simulink model "five_tank_hybrid_system"  (R2019a)
settings: Solver=FixedStepDiscrete  StartTime=0.0  StopTime=T  FixedStep=Ts  RelTol=1e-3
InitFcn:
  | load_parameters
values from neighbouring files (symbols this model uses):
  A1u = 0.0573+0.00286    (= 0.06016)    [load_parameters.m]
  A2u = 0.0573+0.00286    (= 0.06016)    [load_parameters.m]
  A3u = 0.0346+0.0017    (= 0.0363)    [load_parameters.m]
  A4u = 0.0346+0.0017    (= 0.0363)    [load_parameters.m]
  A5u = 0.0707+0.00353    (= 0.07423)    [load_parameters.m]
  Ap1u = 3.167e-5+6.33e-6    (= 3.8e-05)    [load_parameters.m]
  Ap2u = 3.167e-5+6.33e-6    (= 3.8e-05)    [load_parameters.m]
  Ap3u = 3.167e-5+6.33e-6    (= 3.8e-05)    [load_parameters.m]
  Ap4u = 3.167e-5+6.33e-6    (= 3.8e-05)    [load_parameters.m]
  Ap5u = 3.167e-5+6.33e-6    (= 3.8e-05)    [load_parameters.m]
  Av1u = 3.167e-5+6.33e-6    (= 3.8e-05)    [load_parameters.m]
  Av2u = 3.167e-5+6.33e-6    (= 3.8e-05)    [load_parameters.m]
  Av3u = 3.167e-5+6.33e-6    (= 3.8e-05)    [load_parameters.m]
  Av4u = 3.167e-5+6.33e-6    (= 3.8e-05)    [load_parameters.m]
  cp1u = 0.68-0.0675    (= 0.6125)    [load_parameters.m]
  cp2u = 0.68-0.0675    (= 0.6125)    [load_parameters.m]
  cp3u = 0.4-0.038    (= 0.362)    [load_parameters.m]
  cp4u = 0.4-0.038    (= 0.362)    [load_parameters.m]
  cp5u = 0.7-0.068    (= 0.632)    [load_parameters.m]
  cv1u = 0.62-0.0615    (= 0.5585)    [load_parameters.m]
  cv2u = 0.62-0.0615    (= 0.5585)    [load_parameters.m]
  cv3u = 0.37-0.0365    (= 0.3335)    [load_parameters.m]
  cv4u = 0.37-0.0365    (= 0.3335)    [load_parameters.m]
  g = 9.81    [load_parameters.m]
  rho1 = 0.005    [load_parameters.m]
  rho2 = 0.005    [load_parameters.m]
  rho3 = 0.005    [load_parameters.m]
  rho4 = 0.005    [load_parameters.m]
  rho5 = 0.0063    [load_parameters.m]
  Ts = 0.01    [load_parameters.m]
  v = 0.02    [load_parameters.m]
  x1_0 = 0.3    [load_parameters.m]
  X1max = 0.4    [load_parameters.m]
  X1min = 0.1    [load_parameters.m]
  X1overflow = 0.405    [load_parameters.m]
  x2_0 = 0.12    [load_parameters.m]
  X2max = 0.4    [load_parameters.m]
  X2min = 0.1    [load_parameters.m]
  X2overflow = 0.405    [load_parameters.m]
  x3_0 = 0.15    [load_parameters.m]
  X3max = 0.35    [load_parameters.m]
  X3min = 0.1    [load_parameters.m]
  X3overflow = 0.355    [load_parameters.m]
  x4_0 = 0.3    [load_parameters.m]
  X4max = 0.35    [load_parameters.m]
  X4min = 0.1    [load_parameters.m]
  X4overflow = 0.355    [load_parameters.m]
  x5_0 = 0.09    [load_parameters.m]
  X5max = 0.2    [load_parameters.m]
  X5min = 0.05    [load_parameters.m]
  X5overflow = 0.205    [load_parameters.m]
  xi = 0.02    [load_parameters.m]
undefined symbols (not defined in the file or in its folder): dfilt, DiscIntNeverNeededParam
libraries: dsparch4 x5
(part 1 of 2)
settings Model: Creator=Constantinos  LastModifiedBy=Constantinos
settings DataIOCC: ReturnWorkspaceOutputs=off
settings DebuggingCC: PregeneratedLibrarySubsystemCodeDiagnostic=none  ArithmeticOperatorsInVariantConditions=warning
settings SFSimCC: SimUseLocalCustomCode=off
settings RTWCC: RTWUseLocalCustomCode=off

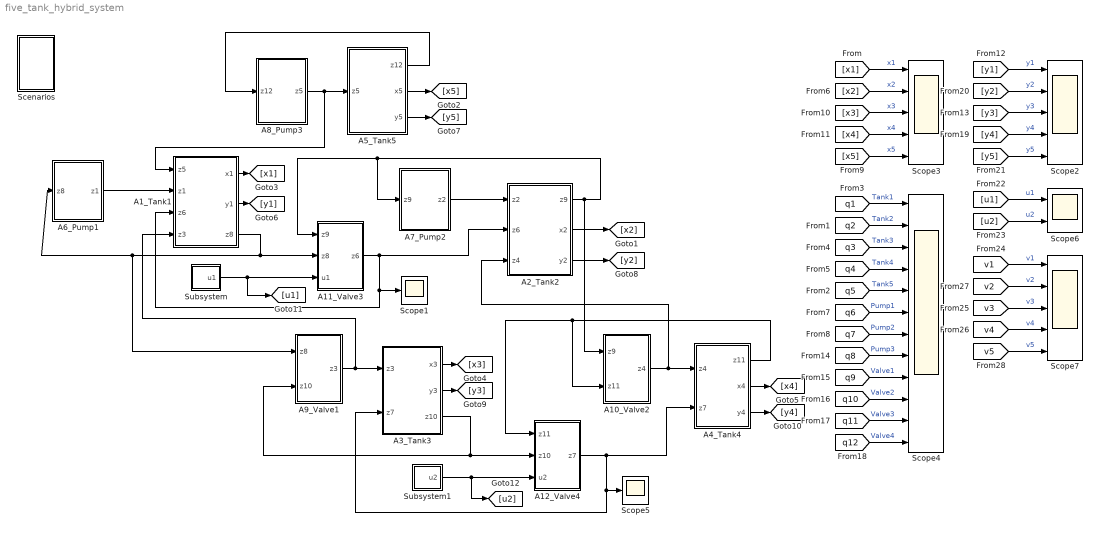
== system five_tank_hybrid_system ==
  A10_Valve2 : Subsystem
  A11_Valve3 : Subsystem
  A12_Valve4 : Subsystem
  A1_Tank1 : Subsystem
  A2_Tank2 : Subsystem
  A3_Tank3 : Subsystem
  A4_Tank4 : Subsystem
  A5_Tank5 : Subsystem
  A6_Pump1 : Subsystem
  A7_Pump2 : Subsystem
  A8_Pump3 : Subsystem
  A9_Valve1 : Subsystem
  Scenarios : Subsystem
  Scope1 : Scope
  Scope2 : Scope  NumInputPorts=5
  Scope3 : Scope  NumInputPorts=5
  Scope4 : Scope  NumInputPorts=12
  Scope5 : Scope
  Scope6 : Scope  NumInputPorts=2
  Scope7 : Scope  NumInputPorts=5
  Subsystem : Subsystem
  Subsystem1 : Subsystem
  wires:
  A6_Pump1/1(z1) -> A1_Tank1/2(z1)
  A7_Pump2/1(z2) -> A2_Tank2/1(z2)
  A8_Pump3/1(z5) -> A1_Tank1/1(z5), A5_Tank5/1(z5)
  A5_Tank5/1(z12) -> A8_Pump3/1(z12)
  A1_Tank1/3(z8) -> A6_Pump1/1(z8), A9_Valve1/1(z8), A11_Valve3/2(z8)
  A11_Valve3/1(z6) -> A2_Tank2/2(z6), Scope1/1, A1_Tank1/3(z6)
  A2_Tank2/1(z9) -> A7_Pump2/1(z9), A11_Valve3/1(z9), A10_Valve2/1(z9)
  A3_Tank3/3(z10) -> A12_Valve4/2(z10), A9_Valve1/2(z10)
  A12_Valve4/1(z7) -> Scope5/1, A3_Tank3/2(z7), A4_Tank4/2(z7)
  A4_Tank4/1(z11) -> A12_Valve4/1(z11), A10_Valve2/2(z11)
  A9_Valve1/1(z3) -> A1_Tank1/4(z3), A3_Tank3/1(z3)
  A10_Valve2/1(z4) -> A2_Tank2/3(z4), A4_Tank4/1(z4)
  A5_Tank5/2(x5) -> [x5]
  [q1] -> Scope4/1  "Tank1"
  [x4] -> Scope3/4  "x4"
  [q6] -> Scope4/6  "Pump1"
  [q4] -> Scope4/4  "Tank4"
  [x2] -> Scope3/2  "x2"
  [q5] -> Scope4/5  "Tank5"
  [q2] -> Scope4/2  "Tank2"
  [q9] -> Scope4/9  "Valve1"
  [q12] -> Scope4/12  "Valve4"
  [q3] -> Scope4/3  "Tank3"
  [x3] -> Scope3/3  "x3"
  [x1] -> Scope3/1  "x1"
  [q10] -> Scope4/10  "Valve2"
  [q8] -> Scope4/8  "Pump3"
  [q11] -> Scope4/11  "Valve3"
  [q7] -> Scope4/7  "Pump2"
  A2_Tank2/2(x2) -> [x2]
  A1_Tank1/1(x1) -> [x1]
  A3_Tank3/1(x3) -> [x3]
  A4_Tank4/2(x4) -> [x4]
  A1_Tank1/2(y1) -> [y1]
  [y1] -> Scope2/1  "y1"
  [y5] -> Scope2/5  "y5"
  [y3] -> Scope2/3  "y3"
  [y2] -> Scope2/2  "y2"
  [y4] -> Scope2/4  "y4"
  A5_Tank5/3(y5) -> [y5]
  A2_Tank2/3(y2) -> [y2]
  A3_Tank3/2(y3) -> [y3]
  A4_Tank4/3(y4) -> [y4]
  [x5] -> Scope3/5  "x5"
  [u1] -> Scope6/1  "u1"
  [u2] -> Scope6/2  "u2"
  [v4] -> Scope7/4  "v4"
  [v2] -> Scope7/2  "v2"
  [v3] -> Scope7/3  "v3"
  [v5] -> Scope7/5  "v5"
  [v1] -> Scope7/1  "v1"
  Subsystem1/1(u2) -> [u2], A12_Valve4/3(u2)
  Subsystem/1(u1) -> [u1], A11_Valve3/3(u1)

== system five_tank_hybrid_system/A10_Valve2 ==
  z9 : Inport
  z11 : Inport  Port=2
  Chart : Stateflow chart  TreatAsAtomicUnit=on
  Constant1 : Constant  Value=0
  Constant3 : Constant  Value=cv2u
  Constant4 : Constant  Value=Av2u
  Constant5 : Constant  Value=g
  Index Vector : MultiPortSwitch  DataPortOrder=Specify indices  Inputs=1  DataPortIndices={1,2,3,4}
  MATLAB Function : MATLAB Function  TreatAsAtomicUnit=on
  z4 : Outport
  tag scope: q10=global
  wires:
  Index Vector/1 -> z4/1
  [phi12] -> Chart/3(phi12)
  [phi11] -> Chart/2(phi11)
  MATLAB Function/1(z) -> Index Vector/3, Index Vector/5
  Constant4/1 -> MATLAB Function/2(Av)
  Constant5/1 -> MATLAB Function/4(g)
  z11/1 -> Chart/1(x4)
  Constant3/1 -> MATLAB Function/1(cv)
  Chart/1(q) -> [q10], Index Vector/1
  Constant1/1 -> Index Vector/4, Index Vector/2
  z9/1 -> MATLAB Function/3(in1)

== system five_tank_hybrid_system/A11_Valve3 ==
  z9 : Inport
  z8 : Inport  Port=2
  u1 : Inport  Port=3
  Chart : Stateflow chart  TreatAsAtomicUnit=on
  Constant1 : Constant  Value=0
  Constant3 : Constant  Value=cv3u
  Constant4 : Constant  Value=Av3u
  Constant5 : Constant  Value=g
  Index Vector : MultiPortSwitch  DataPortOrder=Specify indices  Inputs=1  DataPortIndices={1,2,3,4}
  MATLAB Function : MATLAB Function  TreatAsAtomicUnit=on
  z6 : Outport
  tag scope: q11=global
  wires:
  z9/1 -> MATLAB Function/4(in2)
  Constant3/1 -> MATLAB Function/1(cv)
  z8/1 -> MATLAB Function/3(in1)
  Constant5/1 -> MATLAB Function/5(g)
  Constant4/1 -> MATLAB Function/2(Av)
  MATLAB Function/1(z) -> Index Vector/3, Index Vector/5
  Chart/1(q) -> [q11], Index Vector/1
  [phi13] -> Chart/2(phi13)
  [phi14] -> Chart/3(phi14)
  Index Vector/1 -> z6/1
  u1/1 -> Chart/1(u1)
  Constant1/1 -> Index Vector/4, Index Vector/2

== system five_tank_hybrid_system/A12_Valve4 ==
  z11 : Inport
  z10 : Inport  Port=2
  u2 : Inport  Port=3
  Chart : Stateflow chart  TreatAsAtomicUnit=on
  Constant2 : Constant  Value=0
  Constant3 : Constant  Value=cv4u
  Constant4 : Constant  Value=Av4u
  Constant5 : Constant  Value=g
  Index Vector : MultiPortSwitch  DataPortOrder=Specify indices  Inputs=1  DataPortIndices={1,2,3,4}
  MATLAB Function : MATLAB Function  TreatAsAtomicUnit=on
  z7 : Outport
  tag scope: q12=global
  wires:
  u2/1 -> Chart/1(u2)
  Index Vector/1 -> z7/1
  [phi16] -> Chart/3(phi16)
  [phi15] -> Chart/2(phi15)
  Chart/1(q) -> [q12], Index Vector/1
  MATLAB Function/1(z) -> Index Vector/3, Index Vector/5
  Constant4/1 -> MATLAB Function/2(Av)
  Constant5/1 -> MATLAB Function/5(g)
  Constant2/1 -> Index Vector/2, Index Vector/4
  z10/1 -> MATLAB Function/3(in1)
  Constant3/1 -> MATLAB Function/1(cv)
  z11/1 -> MATLAB Function/4(in2)

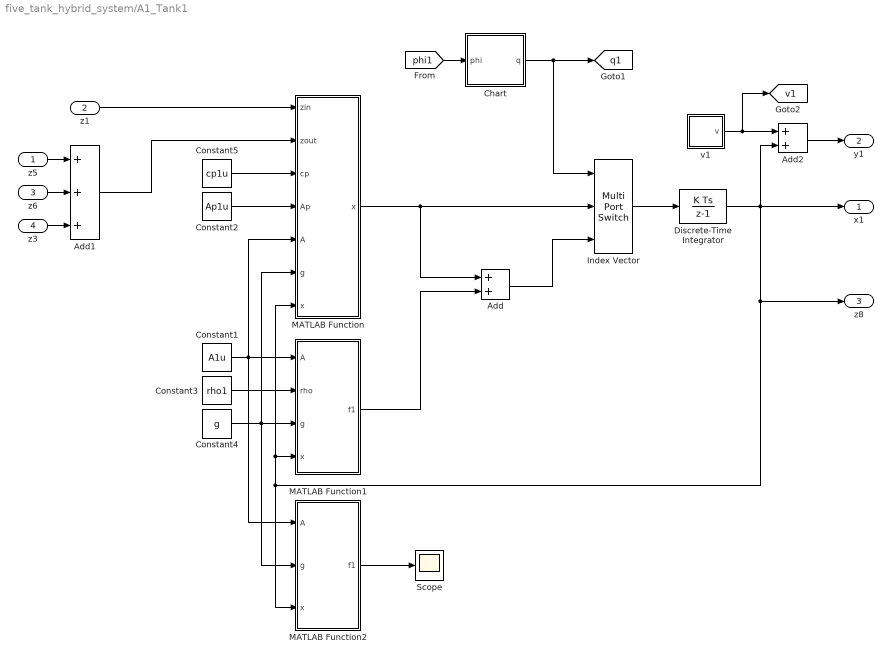
== system five_tank_hybrid_system/A1_Tank1 ==
  z5 : Inport
  z1 : Inport  Port=2
  z6 : Inport  Port=3
  z3 : Inport  Port=4
  Add : Sum
  Add1 : Sum  Inputs=+++
  Add2 : Sum
  Chart : Stateflow chart  TreatAsAtomicUnit=on
  Constant1 : Constant  Value=A1u
  Constant2 : Constant  Value=Ap1u
  Constant3 : Constant  Value=rho1
  Constant4 : Constant  Value=g
  Constant5 : Constant  Value=cp1u
  Discrete-Time Integrator : DiscreteIntegrator  InitialCondition=x1_0  SampleTime=-1  LimitOutput=on  UpperSaturationLimit=X1overflow  LowerSaturationLimit=0  ICPrevOutput=DiscIntNeverNeededParam  ICPrevScaledInput=DiscIntNeverNeededParam
  Index Vector : MultiPortSwitch  DataPortOrder=Specify indices  Inputs=1  DataPortIndices={1,2}
  MATLAB Function : MATLAB Function  TreatAsAtomicUnit=on
  MATLAB Function1 : MATLAB Function  TreatAsAtomicUnit=on
  MATLAB Function2 : MATLAB Function  TreatAsAtomicUnit=on
  Scope : Scope
  v1 : Subsystem
  x1 : Outport
  y1 : Outport  Port=2
  z8 : Outport  Port=3
  tag scope: q1=global, v1=global
  wires:
  Index Vector/1 -> Discrete-Time Integrator/1
  Add/1 -> Index Vector/3
  MATLAB Function/1(x) -> Add/1, Index Vector/2
  MATLAB Function1/1(f1) -> Add/2
  Discrete-Time Integrator/1 -> Add2/2, x1/1, MATLAB Function2/3(x), MATLAB Function/7("x "), MATLAB Function1/4(x), z8/1
  Constant5/1 -> MATLAB Function/3(cp)
  Constant2/1 -> MATLAB Function/4(Ap)
  Constant1/1 -> MATLAB Function2/1(A), MATLAB Function/5(A), MATLAB Function1/1(A)
  Constant3/1 -> MATLAB Function1/2(rho)
  Constant4/1 -> MATLAB Function2/2(g), MATLAB Function/6(g), MATLAB Function1/3(g)
  z1/1 -> MATLAB Function/1(zin)
  z3/1 -> Add1/3
  z6/1 -> Add1/2
  z5/1 -> Add1/1
  Add1/1 -> MATLAB Function/2(zout)
  Chart/1(q) -> [q1], Index Vector/1
  [phi1] -> Chart/1(phi)
  v1/1(v) -> [v1], Add2/1
  Add2/1 -> y1/1
  MATLAB Function2/1(f1) -> Scope/1

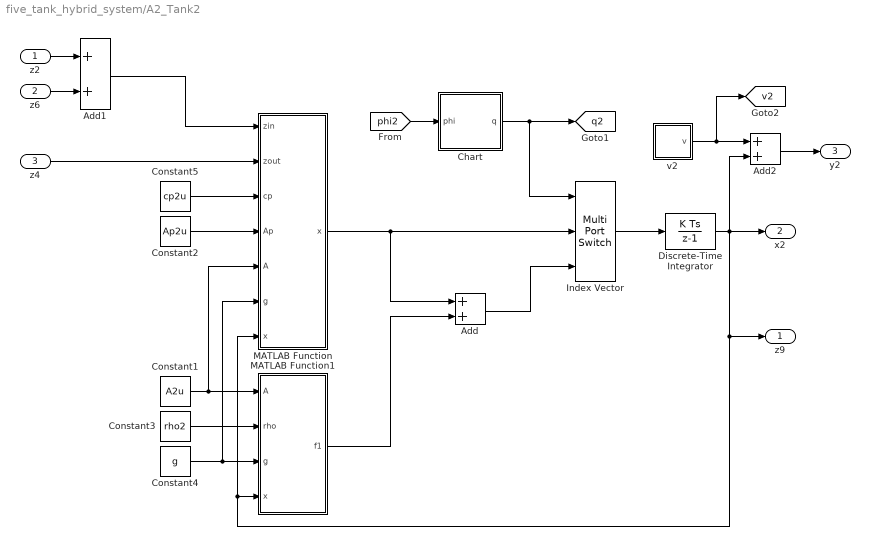
== system five_tank_hybrid_system/A2_Tank2 ==
  z2 : Inport
  z6 : Inport  Port=2
  z4 : Inport  Port=3
  Add : Sum
  Add1 : Sum
  Add2 : Sum
  Chart : Stateflow chart  TreatAsAtomicUnit=on
  Constant1 : Constant  Value=A2u
  Constant2 : Constant  Value=Ap2u
  Constant3 : Constant  Value=rho2
  Constant4 : Constant  Value=g
  Constant5 : Constant  Value=cp2u
  Discrete-Time Integrator : DiscreteIntegrator  InitialCondition=x2_0  SampleTime=-1  LimitOutput=on  UpperSaturationLimit=X2overflow  LowerSaturationLimit=0  ICPrevOutput=DiscIntNeverNeededParam  ICPrevScaledInput=DiscIntNeverNeededParam
  Index Vector : MultiPortSwitch  DataPortOrder=Specify indices  Inputs=1  DataPortIndices={1,2}
  MATLAB Function : MATLAB Function  TreatAsAtomicUnit=on
  MATLAB Function1 : MATLAB Function  TreatAsAtomicUnit=on
  v2 : Subsystem
  z9 : Outport
  x2 : Outport  Port=2
  y2 : Outport  Port=3
  tag scope: q2=global, v2=global
  wires:
  Constant4/1 -> MATLAB Function/6(g), MATLAB Function1/3(g)
  Constant3/1 -> MATLAB Function1/2(rho)
  Constant1/1 -> MATLAB Function1/1(A), MATLAB Function/5(A)
  Constant2/1 -> MATLAB Function/4(Ap)
  Constant5/1 -> MATLAB Function/3(cp)
  MATLAB Function1/1(f1) -> Add/2
  MATLAB Function/1(x) -> Index Vector/2, Add/1
  Add/1 -> Index Vector/3
  Index Vector/1 -> Discrete-Time Integrator/1
  [phi2] -> Chart/1(phi)
  Chart/1(q) -> [q2], Index Vector/1
  Discrete-Time Integrator/1 -> Add2/2, x2/1, z9/1, MATLAB Function/7("x "), MATLAB Function1/4(x)
  Add2/1 -> y2/1
  v2/1(v) -> [v2], Add2/1
  Add1/1 -> MATLAB Function/1(zin)
  z2/1 -> Add1/1
  z6/1 -> Add1/2
  z4/1 -> MATLAB Function/2(zout)

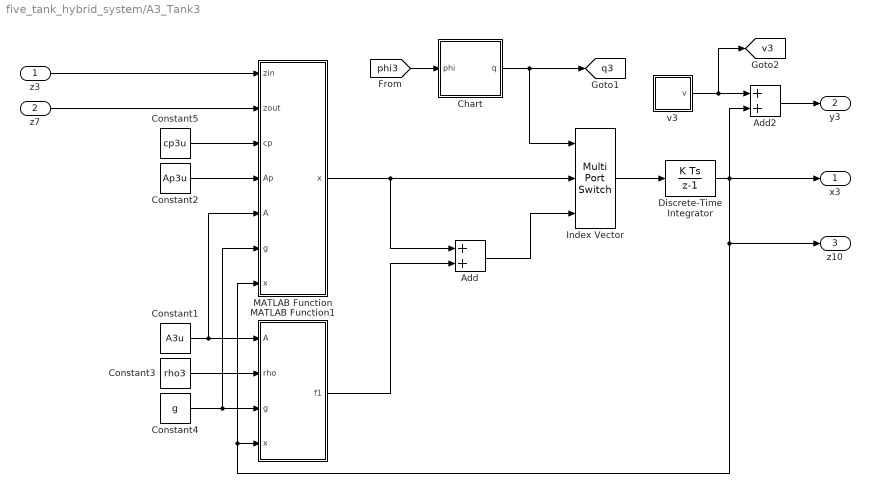
== system five_tank_hybrid_system/A3_Tank3 ==
  z3 : Inport
  z7 : Inport  Port=2
  Add : Sum
  Add2 : Sum
  Chart : Stateflow chart  TreatAsAtomicUnit=on
  Constant1 : Constant  Value=A3u
  Constant2 : Constant  Value=Ap3u
  Constant3 : Constant  Value=rho3
  Constant4 : Constant  Value=g
  Constant5 : Constant  Value=cp3u
  Discrete-Time Integrator : DiscreteIntegrator  InitialCondition=x3_0  SampleTime=-1  LimitOutput=on  UpperSaturationLimit=X3overflow  LowerSaturationLimit=0  ICPrevOutput=DiscIntNeverNeededParam  ICPrevScaledInput=DiscIntNeverNeededParam
  Index Vector : MultiPortSwitch  DataPortOrder=Specify indices  Inputs=1  DataPortIndices={1,2}
  MATLAB Function : MATLAB Function  TreatAsAtomicUnit=on
  MATLAB Function1 : MATLAB Function  TreatAsAtomicUnit=on
  v3 : Subsystem
  x3 : Outport
  y3 : Outport  Port=2
  z10 : Outport  Port=3
  tag scope: q3=global, v3=global
  wires:
  Chart/1(q) -> [q3], Index Vector/1
  [phi3] -> Chart/1(phi)
  Index Vector/1 -> Discrete-Time Integrator/1
  Add/1 -> Index Vector/3
  MATLAB Function/1(x) -> Add/1, Index Vector/2
  MATLAB Function1/1(f1) -> Add/2
  Constant5/1 -> MATLAB Function/3(cp)
  Constant2/1 -> MATLAB Function/4(Ap)
  Constant1/1 -> MATLAB Function/5(A), MATLAB Function1/1(A)
  Constant3/1 -> MATLAB Function1/2(rho)
  Constant4/1 -> MATLAB Function1/3(g), MATLAB Function/6(g)
  z3/1 -> MATLAB Function/1(zin)
  z7/1 -> MATLAB Function/2(zout)
  v3/1(v) -> [v3], Add2/1
  Discrete-Time Integrator/1 -> Add2/2, x3/1, MATLAB Function1/4(x), MATLAB Function/7("x "), z10/1
  Add2/1 -> y3/1

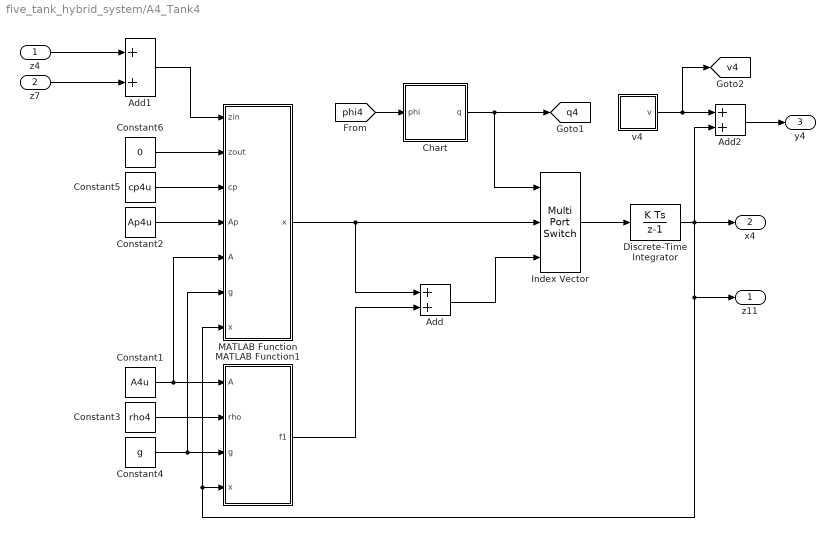
== system five_tank_hybrid_system/A4_Tank4 ==
  z4 : Inport
  z7 : Inport  Port=2
  Add : Sum
  Add1 : Sum
  Add2 : Sum
  Chart : Stateflow chart  TreatAsAtomicUnit=on
  Constant1 : Constant  Value=A4u
  Constant2 : Constant  Value=Ap4u
  Constant3 : Constant  Value=rho4
  Constant4 : Constant  Value=g
  Constant5 : Constant  Value=cp4u
  Constant6 : Constant  Value=0
  Discrete-Time Integrator : DiscreteIntegrator  InitialCondition=x4_0  SampleTime=-1  LimitOutput=on  UpperSaturationLimit=X4overflow  LowerSaturationLimit=0  ICPrevOutput=DiscIntNeverNeededParam  ICPrevScaledInput=DiscIntNeverNeededParam
  Index Vector : MultiPortSwitch  DataPortOrder=Specify indices  Inputs=1  DataPortIndices={1,2}
  MATLAB Function : MATLAB Function  TreatAsAtomicUnit=on
  MATLAB Function1 : MATLAB Function  TreatAsAtomicUnit=on
  v4 : Subsystem
  z11 : Outport
  x4 : Outport  Port=2
  y4 : Outport  Port=3
  tag scope: q4=global, v4=global
  wires:
  z4/1 -> Add1/1
  Constant4/1 -> MATLAB Function/6(g), MATLAB Function1/3(g)
  Constant3/1 -> MATLAB Function1/2(rho)
  Constant1/1 -> MATLAB Function1/1(A), MATLAB Function/5(A)
  Constant2/1 -> MATLAB Function/4(Ap)
  Constant5/1 -> MATLAB Function/3(cp)
  MATLAB Function1/1(f1) -> Add/2
  MATLAB Function/1(x) -> Index Vector/2, Add/1
  Add/1 -> Index Vector/3
  Index Vector/1 -> Discrete-Time Integrator/1
  [phi4] -> Chart/1(phi)
  Chart/1(q) -> [q4], Index Vector/1
  v4/1(v) -> [v4], Add2/1
  Discrete-Time Integrator/1 -> Add2/2, x4/1, MATLAB Function/7("x "), MATLAB Function1/4(x), z11/1
  Add2/1 -> y4/1
  Add1/1 -> MATLAB Function/1(zin)
  z7/1 -> Add1/2
  Constant6/1 -> MATLAB Function/2(zout)

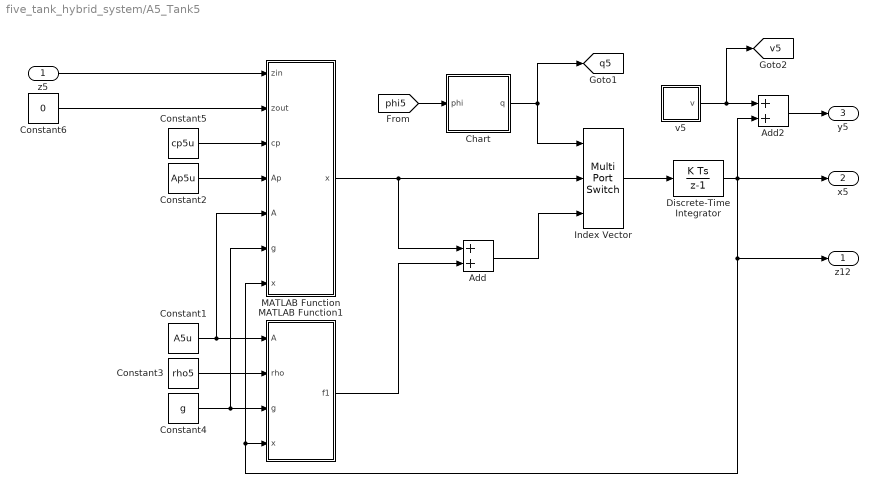
== system five_tank_hybrid_system/A5_Tank5 ==
  z5 : Inport
  Add : Sum
  Add2 : Sum
  Chart : Stateflow chart  TreatAsAtomicUnit=on
  Constant1 : Constant  Value=A5u
  Constant2 : Constant  Value=Ap5u
  Constant3 : Constant  Value=rho5
  Constant4 : Constant  Value=g
  Constant5 : Constant  Value=cp5u
  Constant6 : Constant  Value=0
  Discrete-Time Integrator : DiscreteIntegrator  InitialCondition=x5_0  SampleTime=-1  LimitOutput=on  UpperSaturationLimit=X5overflow  LowerSaturationLimit=0  ICPrevOutput=DiscIntNeverNeededParam  ICPrevScaledInput=DiscIntNeverNeededParam
  Index Vector : MultiPortSwitch  DataPortOrder=Specify indices  Inputs=1  DataPortIndices={1,2}
  MATLAB Function : MATLAB Function  TreatAsAtomicUnit=on
  MATLAB Function1 : MATLAB Function  TreatAsAtomicUnit=on
  v5 : Subsystem
  z12 : Outport
  x5 : Outport  Port=2
  y5 : Outport  Port=3
  tag scope: q5=global, v5=global
  wires:
  Chart/1(q) -> [q5], Index Vector/1
  [phi5] -> Chart/1(phi)
  Index Vector/1 -> Discrete-Time Integrator/1
  Add/1 -> Index Vector/3
  MATLAB Function/1(x) -> Add/1, Index Vector/2
  MATLAB Function1/1(f1) -> Add/2
  Constant5/1 -> MATLAB Function/3(cp)
  Constant2/1 -> MATLAB Function/4(Ap)
  Constant1/1 -> MATLAB Function/5(A), MATLAB Function1/1(A)
  Constant3/1 -> MATLAB Function1/2(rho)
  Constant4/1 -> MATLAB Function1/3(g), MATLAB Function/6(g)
  z5/1 -> MATLAB Function/1(zin)
  Constant6/1 -> MATLAB Function/2(zout)
  Discrete-Time Integrator/1 -> Add2/2, x5/1, z12/1, MATLAB Function1/4(x), MATLAB Function/7("x ")
  Add2/1 -> y5/1
  v5/1(v) -> [v5], Add2/1

== system five_tank_hybrid_system/A6_Pump1 ==
  z8 : Inport
  Chart : Stateflow chart  TreatAsAtomicUnit=on
  Clock : Clock
  Constant : Constant  Value=0
  Fcn : Fcn  Expr=0.5e-5*sin(0.1*u)+1.8e-4
  Index Vector : MultiPortSwitch  DataPortOrder=Specify indices  Inputs=1
  z1 : Outport
  tag scope: q6=global
  wires:
  [phi6] -> Chart/2(phi6)
  Clock/1 -> Fcn/1
  z8/1 -> Chart/1(x1)
  Fcn/1 -> Index Vector/3
  Constant/1 -> Index Vector/4, Index Vector/2
  Chart/1(q) -> [q6], Index Vector/1
  Index Vector/1 -> z1/1

== system five_tank_hybrid_system/A7_Pump2 ==
  z9 : Inport
  Chart1 : Stateflow chart  TreatAsAtomicUnit=on
  Clock1 : Clock
  Constant1 : Constant  Value=0
  Fcn1 : Fcn  Expr=0.5e-5*sin(0.1*u)+1.8e-4
  Index Vector1 : MultiPortSwitch  DataPortOrder=Specify indices  Inputs=1
  z2 : Outport
  tag scope: q7=global
  wires:
  Clock1/1 -> Fcn1/1
  [phi7] -> Chart1/2(phi7)
  z9/1 -> Chart1/1(x2)
  Constant1/1 -> Index Vector1/4, Index Vector1/2
  Fcn1/1 -> Index Vector1/3
  Index Vector1/1 -> z2/1
  Chart1/1(q) -> [q7], Index Vector1/1

== system five_tank_hybrid_system/A8_Pump3 ==
  z12 : Inport
  Chart2 : Stateflow chart  TreatAsAtomicUnit=on
  Clock1 : Clock
  Constant1 : Constant  Value=0
  Fcn1 : Fcn  Expr=0.5e-5*sin(0.1*u)+0.85e-4
  Index Vector1 : MultiPortSwitch  DataPortOrder=Specify indices  Inputs=1
  z5 : Outport
  tag scope: q8=global
  wires:
  Index Vector1/1 -> z5/1
  [phi8] -> Chart2/2(phi8)
  Chart2/1(q) -> [q8], Index Vector1/1
  z12/1 -> Chart2/1(x5)
  Constant1/1 -> Index Vector1/4, Index Vector1/2
  Fcn1/1 -> Index Vector1/3
  Clock1/1 -> Fcn1/1

== system five_tank_hybrid_system/A9_Valve1 ==
  z8 : Inport
  z10 : Inport  Port=2
  Chart : Stateflow chart  TreatAsAtomicUnit=on
  Constant1 : Constant  Value=0
  Constant3 : Constant  Value=cv1u
  Constant4 : Constant  Value=Av1u
  Constant5 : Constant  Value=g
  Index Vector : MultiPortSwitch  DataPortOrder=Specify indices  Inputs=1  DataPortIndices={1,2,3,4}
  MATLAB Function : MATLAB Function  TreatAsAtomicUnit=on
  z3 : Outport
  tag scope: q9=global
  wires:
  Constant3/1 -> MATLAB Function/1(cv)
  z10/1 -> Chart/1(x3)
  Constant5/1 -> MATLAB Function/4(g)
  Constant4/1 -> MATLAB Function/2(Av)
  MATLAB Function/1(z) -> Index Vector/3, Index Vector/5
  Chart/1(q) -> [q9], Index Vector/1
  [phi9] -> Chart/2(phi9)
  [phi10] -> Chart/3(phi10)
  Index Vector/1 -> z3/1
  Constant1/1 -> Index Vector/4, Index Vector/2
  z8/1 -> MATLAB Function/3(in1)

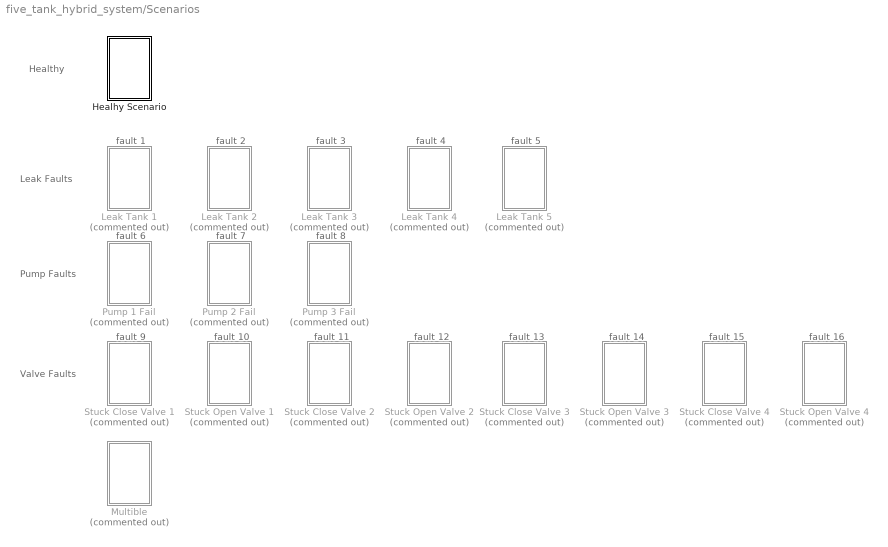
== system five_tank_hybrid_system/Scenarios ==
  note: fault 1
  note: Healthy
  note: Leak Faults
  note: Pump Faults
  note: Valve Faults
  note: fault 2
  note: fault 3
  note: fault 4
  note: fault 5
  note: fault 6
  note: fault 7
  note: fault 8
  note: fault 9
  note: fault 13
  note: fault 10
  note: fault 14
  note: fault 11
  note: fault 15
  note: fault 12
  note: fault 16
  Healhy Scenario : Subsystem
  Leak Tank 1 : Subsystem  Commented=on
  Leak Tank 2 : Subsystem  Commented=on
  Leak Tank 3 : Subsystem  Commented=on
  Leak Tank 4 : Subsystem  Commented=on
  Leak Tank 5 : Subsystem  Commented=on
  Multible : Subsystem  Commented=on
  Pump 1 Fail : Subsystem  Commented=on
  Pump 2 Fail : Subsystem  Commented=on
  Pump 3 Fail : Subsystem  Commented=on
  Stuck Close Valve 1 : Subsystem  Commented=on
  Stuck Close Valve 2 : Subsystem  Commented=on
  Stuck Close Valve 3 : Subsystem  Commented=on
  Stuck Close Valve 4 : Subsystem  Commented=on
  Stuck Open Valve 1 : Subsystem  Commented=on
  Stuck Open Valve 2 : Subsystem  Commented=on
  Stuck Open Valve 3 : Subsystem  Commented=on
  Stuck Open Valve 4 : Subsystem  Commented=on

== system five_tank_hybrid_system/Subsystem ==
  Chart : Stateflow chart  TreatAsAtomicUnit=on
  u1 : Outport
  wires:
  Chart/1(u1) -> u1/1

== system five_tank_hybrid_system/Subsystem1 ==
  Chart : Stateflow chart  TreatAsAtomicUnit=on
  u2 : Outport
  wires:
  Chart/1(u2) -> u2/1

== system five_tank_hybrid_system/A1_Tank1/v1 ==
  Highpass085 : dsparch4/Biquad Filter  Tag=BlockMethodSubSystem  FilterSource=Dialog parameters  CoeffSource=Specify via dialog  FilterObject=dfilt.df2tsos([1 0.3 0.4],[1 0.1 0.2])  IIRFiltStruct=Direct form II  BiQuadCoeffs=[1 -2 1 1 1.6638470300298394 0.8673791772124948;1 -2 1 1 1.4774912143044396 0.65822715568812495;1 -2 1 1 1.3489677452527944 0.51398189421967577;1 -2 1 1 1.2687805392030125 0.42398568894741273;1 -2 1 1 1.2303311697764827 0.38083295281952212]  ScaleValues=[0.050883036795663916;0.045183985345921322;0.041253537241720324;0.038801287436100056;0.037625445760759803;1]  IC=0  ICnum=0  ICden=0  a0Flag=Warning  optimizeScaleValues=on  ScaleValueMode=Specify via input port (g)  InputProcessing=Columns as channels (frame based)  roundingMode=Floor  overflowMode=off  scaleValueFracLength=14  denProdOutputFracLength=30  denAccumFracLength=30  secondMemoryFracLength=15
      settings: SourceProductName=DSP System Toolbox
  Saturation : Saturate  UpperLimit=xi  LowerLimit=-xi
  Scope1 : Scope
  Scope2 : Scope
  noise : UniformRandomNumber  Minimum=-v  Maximum=v  Seed=15  SampleTime=Ts
  v : Outport
  wires:
  noise/1 -> Scope1/1, Highpass085/1
  Highpass085/1 -> Scope2/1, Saturation/1
  Saturation/1 -> v/1

== system five_tank_hybrid_system/A2_Tank2/v2 ==
  Highpass085 : dsparch4/Biquad Filter  Tag=BlockMethodSubSystem  FilterSource=Dialog parameters  CoeffSource=Specify via dialog  FilterObject=dfilt.df2tsos([1 0.3 0.4],[1 0.1 0.2])  IIRFiltStruct=Direct form II  BiQuadCoeffs=[1 -2 1 1 1.6638470300298394 0.8673791772124948;1 -2 1 1 1.4774912143044396 0.65822715568812495;1 -2 1 1 1.3489677452527944 0.51398189421967577;1 -2 1 1 1.2687805392030125 0.42398568894741273;1 -2 1 1 1.2303311697764827 0.38083295281952212]  ScaleValues=[0.050883036795663916;0.045183985345921322;0.041253537241720324;0.038801287436100056;0.037625445760759803;1]  IC=0  ICnum=0  ICden=0  a0Flag=Warning  optimizeScaleValues=on  ScaleValueMode=Specify via input port (g)  InputProcessing=Columns as channels (frame based)  roundingMode=Floor  overflowMode=off  scaleValueFracLength=14  denProdOutputFracLength=30  denAccumFracLength=30  secondMemoryFracLength=15
      settings: SourceProductName=DSP System Toolbox
  Saturation : Saturate  UpperLimit=xi  LowerLimit=-xi
  Scope1 : Scope
  Scope2 : Scope
  noise : UniformRandomNumber  Minimum=-v  Maximum=v  Seed=11  SampleTime=Ts
  v : Outport
  wires:
  noise/1 -> Scope1/1, Highpass085/1
  Highpass085/1 -> Scope2/1, Saturation/1
  Saturation/1 -> v/1

== system five_tank_hybrid_system/A3_Tank3/v3 ==
  Highpass085 : dsparch4/Biquad Filter  Tag=BlockMethodSubSystem  FilterSource=Dialog parameters  CoeffSource=Specify via dialog  FilterObject=dfilt.df2tsos([1 0.3 0.4],[1 0.1 0.2])  IIRFiltStruct=Direct form II  BiQuadCoeffs=[1 -2 1 1 1.6638470300298394 0.8673791772124948;1 -2 1 1 1.4774912143044396 0.65822715568812495;1 -2 1 1 1.3489677452527944 0.51398189421967577;1 -2 1 1 1.2687805392030125 0.42398568894741273;1 -2 1 1 1.2303311697764827 0.38083295281952212]  ScaleValues=[0.050883036795663916;0.045183985345921322;0.041253537241720324;0.038801287436100056;0.037625445760759803;1]  IC=0  ICnum=0  ICden=0  a0Flag=Warning  optimizeScaleValues=on  ScaleValueMode=Specify via input port (g)  InputProcessing=Columns as channels (frame based)  roundingMode=Floor  overflowMode=off  scaleValueFracLength=14  denProdOutputFracLength=30  denAccumFracLength=30  secondMemoryFracLength=15
      settings: SourceProductName=DSP System Toolbox
  Saturation : Saturate  UpperLimit=xi  LowerLimit=-xi
  Scope1 : Scope
  Scope2 : Scope
  noise : UniformRandomNumber  Minimum=-v  Maximum=v  Seed=7  SampleTime=Ts
  v : Outport
  wires:
  noise/1 -> Scope1/1, Highpass085/1
  Highpass085/1 -> Scope2/1, Saturation/1
  Saturation/1 -> v/1

== system five_tank_hybrid_system/A4_Tank4/v4 ==
  Highpass085 : dsparch4/Biquad Filter  Tag=BlockMethodSubSystem  FilterSource=Dialog parameters  CoeffSource=Specify via dialog  FilterObject=dfilt.df2tsos([1 0.3 0.4],[1 0.1 0.2])  IIRFiltStruct=Direct form II  BiQuadCoeffs=[1 -2 1 1 1.6638470300298394 0.8673791772124948;1 -2 1 1 1.4774912143044396 0.65822715568812495;1 -2 1 1 1.3489677452527944 0.51398189421967577;1 -2 1 1 1.2687805392030125 0.42398568894741273;1 -2 1 1 1.2303311697764827 0.38083295281952212]  ScaleValues=[0.050883036795663916;0.045183985345921322;0.041253537241720324;0.038801287436100056;0.037625445760759803;1]  IC=0  ICnum=0  ICden=0  a0Flag=Warning  optimizeScaleValues=on  ScaleValueMode=Specify via input port (g)  InputProcessing=Columns as channels (frame based)  roundingMode=Floor  overflowMode=off  scaleValueFracLength=14  denProdOutputFracLength=30  denAccumFracLength=30  secondMemoryFracLength=15
      settings: SourceProductName=DSP System Toolbox
  Saturation : Saturate  UpperLimit=xi  LowerLimit=-xi
  Scope1 : Scope
  Scope2 : Scope
  noise : UniformRandomNumber  Minimum=-v  Maximum=v  Seed=18  SampleTime=Ts
  v : Outport
  wires:
  noise/1 -> Scope1/1, Highpass085/1
  Highpass085/1 -> Scope2/1, Saturation/1
  Saturation/1 -> v/1

== system five_tank_hybrid_system/A5_Tank5/v5 ==
  Highpass085 : dsparch4/Biquad Filter  Tag=BlockMethodSubSystem  FilterSource=Dialog parameters  CoeffSource=Specify via dialog  FilterObject=dfilt.df2tsos([1 0.3 0.4],[1 0.1 0.2])  IIRFiltStruct=Direct form II  BiQuadCoeffs=[1 -2 1 1 1.6638470300298394 0.8673791772124948;1 -2 1 1 1.4774912143044396 0.65822715568812495;1 -2 1 1 1.3489677452527944 0.51398189421967577;1 -2 1 1 1.2687805392030125 0.42398568894741273;1 -2 1 1 1.2303311697764827 0.38083295281952212]  ScaleValues=[0.050883036795663916;0.045183985345921322;0.041253537241720324;0.038801287436100056;0.037625445760759803;1]  IC=0  ICnum=0  ICden=0  a0Flag=Warning  optimizeScaleValues=on  ScaleValueMode=Specify via input port (g)  InputProcessing=Columns as channels (frame based)  roundingMode=Floor  overflowMode=off  scaleValueFracLength=14  denProdOutputFracLength=30  denAccumFracLength=30  secondMemoryFracLength=15
      settings: SourceProductName=DSP System Toolbox
  Saturation : Saturate  UpperLimit=xi  LowerLimit=-xi
  Scope1 : Scope
  Scope2 : Scope
  noise : UniformRandomNumber  Minimum=-v  Maximum=v  Seed=15  SampleTime=Ts
  v : Outport
  wires:
  noise/1 -> Scope1/1, Highpass085/1
  Highpass085/1 -> Scope2/1, Saturation/1
  Saturation/1 -> v/1

== system five_tank_hybrid_system/Scenarios/Healhy Scenario ==
  Healthy : Stateflow chart  TreatAsAtomicUnit=on
  tag scope: phi10=global, phi11=global, phi12=global, phi13=global, phi14=global, phi15=global, phi16=global, phi1=global, phi2=global, phi3=global, phi4=global, phi5=global, phi6=global, phi7=global, phi8=global, phi9=global
  wires:
  Healthy/16(phi16) -> [phi16]
  Healthy/15(phi15) -> [phi15]
  Healthy/1(phi1) -> [phi1]
  Healthy/2(phi2) -> [phi2]
  Healthy/3(phi3) -> [phi3]
  Healthy/4(phi4) -> [phi4]
  Healthy/5(phi5) -> [phi5]
  Healthy/6(phi6) -> [phi6]
  Healthy/7(phi7) -> [phi7]
  Healthy/8(phi8) -> [phi8]
  Healthy/9(phi9) -> [phi9]
  Healthy/10(phi10) -> [phi10]
  Healthy/11(phi11) -> [phi11]
  Healthy/12(phi12) -> [phi12]
  Healthy/13(phi13) -> [phi13]
  Healthy/14(phi14) -> [phi14]

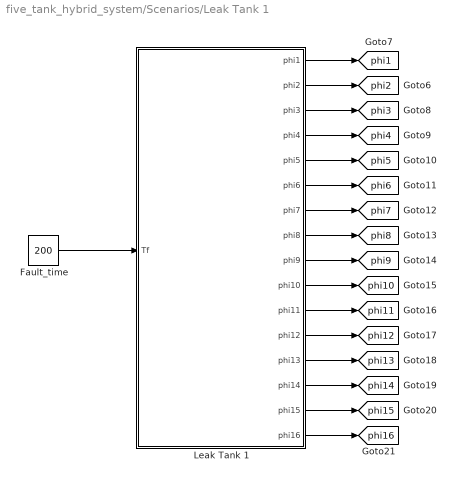
== system five_tank_hybrid_system/Scenarios/Leak Tank 1 ==
  Fault_time : Constant  Value=200
  Leak Tank 1 : Stateflow chart  TreatAsAtomicUnit=on
  tag scope: phi10=global, phi11=global, phi12=global, phi13=global, phi14=global, phi15=global, phi16=global, phi1=global, phi2=global, phi3=global, phi4=global, phi5=global, phi6=global, phi7=global, phi8=global, phi9=global
  wires:
  Leak Tank 1/14(phi14) -> [phi14]
  Leak Tank 1/13(phi13) -> [phi13]
  Leak Tank 1/12(phi12) -> [phi12]
  Leak Tank 1/11(phi11) -> [phi11]
  Leak Tank 1/10(phi10) -> [phi10]
  Leak Tank 1/9(phi9) -> [phi9]
  Leak Tank 1/8(phi8) -> [phi8]
  Leak Tank 1/7(phi7) -> [phi7]
  Leak Tank 1/6(phi6) -> [phi6]
  Leak Tank 1/5(phi5) -> [phi5]
  Leak Tank 1/4(phi4) -> [phi4]
  Leak Tank 1/3(phi3) -> [phi3]
  Leak Tank 1/2(phi2) -> [phi2]
  Leak Tank 1/1(phi1) -> [phi1]
  Leak Tank 1/15(phi15) -> [phi15]
  Leak Tank 1/16(phi16) -> [phi16]
  Fault_time/1 -> Leak Tank 1/1(Tf)

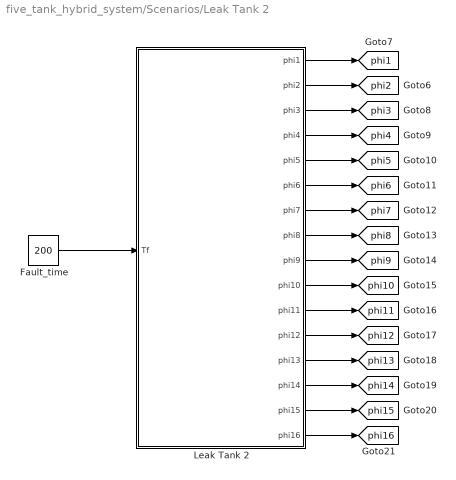
== system five_tank_hybrid_system/Scenarios/Leak Tank 2 ==
  Fault_time : Constant  Value=200
  Leak Tank 2 : Stateflow chart  TreatAsAtomicUnit=on
  tag scope: phi10=global, phi11=global, phi12=global, phi13=global, phi14=global, phi15=global, phi16=global, phi1=global, phi2=global, phi3=global, phi4=global, phi5=global, phi6=global, phi7=global, phi8=global, phi9=global
  wires:
  Fault_time/1 -> Leak Tank 2/1(Tf)
  Leak Tank 2/16(phi16) -> [phi16]
  Leak Tank 2/15(phi15) -> [phi15]
  Leak Tank 2/1(phi1) -> [phi1]
  Leak Tank 2/2(phi2) -> [phi2]
  Leak Tank 2/3(phi3) -> [phi3]
  Leak Tank 2/4(phi4) -> [phi4]
  Leak Tank 2/5(phi5) -> [phi5]
  Leak Tank 2/6(phi6) -> [phi6]
  Leak Tank 2/7(phi7) -> [phi7]
  Leak Tank 2/8(phi8) -> [phi8]
  Leak Tank 2/9(phi9) -> [phi9]
  Leak Tank 2/10(phi10) -> [phi10]
  Leak Tank 2/11(phi11) -> [phi11]
  Leak Tank 2/12(phi12) -> [phi12]
  Leak Tank 2/13(phi13) -> [phi13]
  Leak Tank 2/14(phi14) -> [phi14]

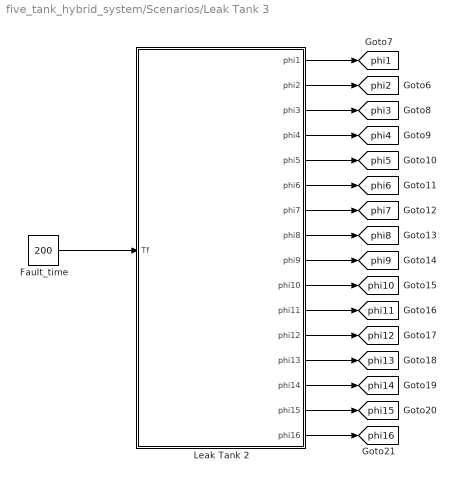
== system five_tank_hybrid_system/Scenarios/Leak Tank 3 ==
  Fault_time : Constant  Value=200
  Leak Tank 2 : Stateflow chart  TreatAsAtomicUnit=on
  tag scope: phi10=global, phi11=global, phi12=global, phi13=global, phi14=global, phi15=global, phi16=global, phi1=global, phi2=global, phi3=global, phi4=global, phi5=global, phi6=global, phi7=global, phi8=global, phi9=global
  wires:
  Fault_time/1 -> Leak Tank 2/1(Tf)
  Leak Tank 2/16(phi16) -> [phi16]
  Leak Tank 2/15(phi15) -> [phi15]
  Leak Tank 2/1(phi1) -> [phi1]
  Leak Tank 2/2(phi2) -> [phi2]
  Leak Tank 2/3(phi3) -> [phi3]
  Leak Tank 2/4(phi4) -> [phi4]
  Leak Tank 2/5(phi5) -> [phi5]
  Leak Tank 2/6(phi6) -> [phi6]
  Leak Tank 2/7(phi7) -> [phi7]
  Leak Tank 2/8(phi8) -> [phi8]
  Leak Tank 2/9(phi9) -> [phi9]
  Leak Tank 2/10(phi10) -> [phi10]
  Leak Tank 2/11(phi11) -> [phi11]
  Leak Tank 2/12(phi12) -> [phi12]
  Leak Tank 2/13(phi13) -> [phi13]
  Leak Tank 2/14(phi14) -> [phi14]

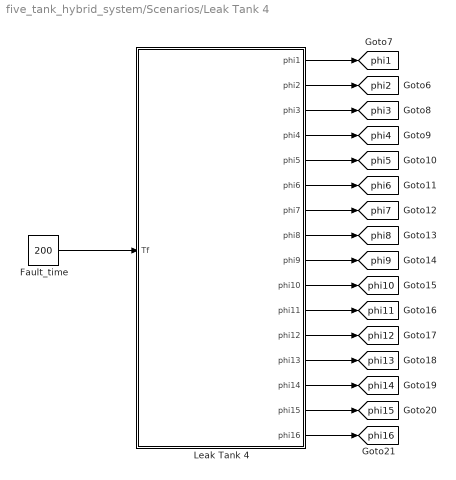
== system five_tank_hybrid_system/Scenarios/Leak Tank 4 ==
  Fault_time : Constant  Value=200
  Leak Tank 4 : Stateflow chart  TreatAsAtomicUnit=on
  tag scope: phi10=global, phi11=global, phi12=global, phi13=global, phi14=global, phi15=global, phi16=global, phi1=global, phi2=global, phi3=global, phi4=global, phi5=global, phi6=global, phi7=global, phi8=global, phi9=global
  wires:
  Fault_time/1 -> Leak Tank 4/1(Tf)
  Leak Tank 4/16(phi16) -> [phi16]
  Leak Tank 4/15(phi15) -> [phi15]
  Leak Tank 4/1(phi1) -> [phi1]
  Leak Tank 4/2(phi2) -> [phi2]
  Leak Tank 4/3(phi3) -> [phi3]
  Leak Tank 4/4(phi4) -> [phi4]
  Leak Tank 4/5(phi5) -> [phi5]
  Leak Tank 4/6(phi6) -> [phi6]
  Leak Tank 4/7(phi7) -> [phi7]
  Leak Tank 4/8(phi8) -> [phi8]
  Leak Tank 4/9(phi9) -> [phi9]
  Leak Tank 4/10(phi10) -> [phi10]
  Leak Tank 4/11(phi11) -> [phi11]
  Leak Tank 4/12(phi12) -> [phi12]
  Leak Tank 4/13(phi13) -> [phi13]
  Leak Tank 4/14(phi14) -> [phi14]

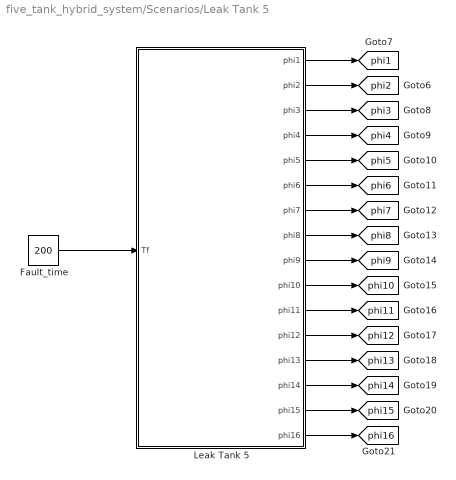
== system five_tank_hybrid_system/Scenarios/Leak Tank 5 ==
  Fault_time : Constant  Value=200
  Leak Tank 5 : Stateflow chart  TreatAsAtomicUnit=on
  tag scope: phi10=global, phi11=global, phi12=global, phi13=global, phi14=global, phi15=global, phi16=global, phi1=global, phi2=global, phi3=global, phi4=global, phi5=global, phi6=global, phi7=global, phi8=global, phi9=global
  wires:
  Leak Tank 5/14(phi14) -> [phi14]
  Leak Tank 5/13(phi13) -> [phi13]
  Leak Tank 5/12(phi12) -> [phi12]
  Leak Tank 5/11(phi11) -> [phi11]
  Leak Tank 5/10(phi10) -> [phi10]
  Leak Tank 5/9(phi9) -> [phi9]
  Leak Tank 5/8(phi8) -> [phi8]
  Leak Tank 5/7(phi7) -> [phi7]
  Leak Tank 5/6(phi6) -> [phi6]
  Leak Tank 5/5(phi5) -> [phi5]
  Leak Tank 5/4(phi4) -> [phi4]
  Leak Tank 5/3(phi3) -> [phi3]
  Leak Tank 5/2(phi2) -> [phi2]
  Leak Tank 5/1(phi1) -> [phi1]
  Leak Tank 5/15(phi15) -> [phi15]
  Leak Tank 5/16(phi16) -> [phi16]
  Fault_time/1 -> Leak Tank 5/1(Tf)

== system five_tank_hybrid_system/Scenarios/Multible ==
  Fault_time : Constant  Value=100
  Stuck Close : Stateflow chart  TreatAsAtomicUnit=on
  tag scope: phi10=global, phi11=global, phi12=global, phi13=global, phi14=global, phi15=global, phi16=global, phi1=global, phi2=global, phi3=global, phi4=global, phi5=global, phi6=global, phi7=global, phi8=global, phi9=global
  wires:
  Fault_time/1 -> Stuck Close/1(Tf)
  Stuck Close/16(phi16) -> [phi16]
  Stuck Close/15(phi15) -> [phi15]
  Stuck Close/1(phi1) -> [phi1]
  Stuck Close/2(phi2) -> [phi2]
  Stuck Close/3(phi3) -> [phi3]
  Stuck Close/4(phi4) -> [phi4]
  Stuck Close/5(phi5) -> [phi5]
  Stuck Close/6(phi6) -> [phi6]
  Stuck Close/7(phi7) -> [phi7]
  Stuck Close/8(phi8) -> [phi8]
  Stuck Close/9(phi9) -> [phi9]
  Stuck Close/10(phi10) -> [phi10]
  Stuck Close/11(phi11) -> [phi11]
  Stuck Close/12(phi12) -> [phi12]
  Stuck Close/13(phi13) -> [phi13]
  Stuck Close/14(phi14) -> [phi14]

== system five_tank_hybrid_system/Scenarios/Pump 1 Fail ==
  Fault_time : Constant  Value=350
  Pump 1 Fail : Stateflow chart  TreatAsAtomicUnit=on
  tag scope: phi10=global, phi11=global, phi12=global, phi13=global, phi14=global, phi15=global, phi16=global, phi1=global, phi2=global, phi3=global, phi4=global, phi5=global, phi6=global, phi7=global, phi8=global, phi9=global
  wires:
  Fault_time/1 -> Pump 1 Fail/1(Tf)
  Pump 1 Fail/16(phi16) -> [phi16]
  Pump 1 Fail/15(phi15) -> [phi15]
  Pump 1 Fail/1(phi1) -> [phi1]
  Pump 1 Fail/2(phi2) -> [phi2]
  Pump 1 Fail/3(phi3) -> [phi3]
  Pump 1 Fail/4(phi4) -> [phi4]
  Pump 1 Fail/5(phi5) -> [phi5]
  Pump 1 Fail/6(phi6) -> [phi6]
  Pump 1 Fail/7(phi7) -> [phi7]
  Pump 1 Fail/8(phi8) -> [phi8]
  Pump 1 Fail/9(phi9) -> [phi9]
  Pump 1 Fail/10(phi10) -> [phi10]
  Pump 1 Fail/11(phi11) -> [phi11]
  Pump 1 Fail/12(phi12) -> [phi12]
  Pump 1 Fail/13(phi13) -> [phi13]
  Pump 1 Fail/14(phi14) -> [phi14]

== system five_tank_hybrid_system/Scenarios/Pump 2 Fail ==
  Fault_time : Constant  Value=350
  Pump 2 Fail : Stateflow chart  TreatAsAtomicUnit=on
  tag scope: phi10=global, phi11=global, phi12=global, phi13=global, phi14=global, phi15=global, phi16=global, phi1=global, phi2=global, phi3=global, phi4=global, phi5=global, phi6=global, phi7=global, phi8=global, phi9=global
  wires:
  Pump 2 Fail/14(phi14) -> [phi14]
  Pump 2 Fail/13(phi13) -> [phi13]
  Pump 2 Fail/12(phi12) -> [phi12]
  Pump 2 Fail/11(phi11) -> [phi11]
  Pump 2 Fail/10(phi10) -> [phi10]
  Pump 2 Fail/9(phi9) -> [phi9]
  Pump 2 Fail/8(phi8) -> [phi8]
  Pump 2 Fail/7(phi7) -> [phi7]
  Pump 2 Fail/6(phi6) -> [phi6]
  Pump 2 Fail/5(phi5) -> [phi5]
  Pump 2 Fail/4(phi4) -> [phi4]
  Pump 2 Fail/3(phi3) -> [phi3]
  Pump 2 Fail/2(phi2) -> [phi2]
  Pump 2 Fail/1(phi1) -> [phi1]
  Pump 2 Fail/15(phi15) -> [phi15]
  Pump 2 Fail/16(phi16) -> [phi16]
  Fault_time/1 -> Pump 2 Fail/1(Tf)

== system five_tank_hybrid_system/Scenarios/Pump 3 Fail ==
  Fault_time : Constant  Value=350
  Pump 3 Fail : Stateflow chart  TreatAsAtomicUnit=on
  tag scope: phi10=global, phi11=global, phi12=global, phi13=global, phi14=global, phi15=global, phi16=global, phi1=global, phi2=global, phi3=global, phi4=global, phi5=global, phi6=global, phi7=global, phi8=global, phi9=global
  wires:
  Fault_time/1 -> Pump 3 Fail/1(Tf)
  Pump 3 Fail/16(phi16) -> [phi16]
  Pump 3 Fail/15(phi15) -> [phi15]
  Pump 3 Fail/1(phi1) -> [phi1]
  Pump 3 Fail/2(phi2) -> [phi2]
  Pump 3 Fail/3(phi3) -> [phi3]
  Pump 3 Fail/4(phi4) -> [phi4]
  Pump 3 Fail/5(phi5) -> [phi5]
  Pump 3 Fail/6(phi6) -> [phi6]
  Pump 3 Fail/7(phi7) -> [phi7]
  Pump 3 Fail/8(phi8) -> [phi8]
  Pump 3 Fail/9(phi9) -> [phi9]
  Pump 3 Fail/10(phi10) -> [phi10]
  Pump 3 Fail/11(phi11) -> [phi11]
  Pump 3 Fail/12(phi12) -> [phi12]
  Pump 3 Fail/13(phi13) -> [phi13]
  Pump 3 Fail/14(phi14) -> [phi14]

== system five_tank_hybrid_system/Scenarios/Stuck Close Valve 1 ==
  Fault_time : Constant  Value=200
  Stuck Close : Stateflow chart  TreatAsAtomicUnit=on
  tag scope: phi10=global, phi11=global, phi12=global, phi13=global, phi14=global, phi15=global, phi16=global, phi1=global, phi2=global, phi3=global, phi4=global, phi5=global, phi6=global, phi7=global, phi8=global, phi9=global
  wires:
  Stuck Close/14(phi14) -> [phi14]
  Stuck Close/13(phi13) -> [phi13]
  Stuck Close/12(phi12) -> [phi12]
  Stuck Close/11(phi11) -> [phi11]
  Stuck Close/10(phi10) -> [phi10]
  Stuck Close/9(phi9) -> [phi9]
  Stuck Close/8(phi8) -> [phi8]
  Stuck Close/7(phi7) -> [phi7]
  Stuck Close/6(phi6) -> [phi6]
  Stuck Close/5(phi5) -> [phi5]
  Stuck Close/4(phi4) -> [phi4]
  Stuck Close/3(phi3) -> [phi3]
  Stuck Close/2(phi2) -> [phi2]
  Stuck Close/1(phi1) -> [phi1]
  Stuck Close/15(phi15) -> [phi15]
  Stuck Close/16(phi16) -> [phi16]
  Fault_time/1 -> Stuck Close/1(Tf)

== system five_tank_hybrid_system/Scenarios/Stuck Close Valve 2 ==
  Fault_time : Constant  Value=400
  Stuck Close : Stateflow chart  TreatAsAtomicUnit=on
  tag scope: phi10=global, phi11=global, phi12=global, phi13=global, phi14=global, phi15=global, phi16=global, phi1=global, phi2=global, phi3=global, phi4=global, phi5=global, phi6=global, phi7=global, phi8=global, phi9=global
  wires:
  Fault_time/1 -> Stuck Close/1(Tf)
  Stuck Close/16(phi16) -> [phi16]
  Stuck Close/15(phi15) -> [phi15]
  Stuck Close/1(phi1) -> [phi1]
  Stuck Close/2(phi2) -> [phi2]
  Stuck Close/3(phi3) -> [phi3]
  Stuck Close/4(phi4) -> [phi4]
  Stuck Close/5(phi5) -> [phi5]
  Stuck Close/6(phi6) -> [phi6]
  Stuck Close/7(phi7) -> [phi7]
  Stuck Close/8(phi8) -> [phi8]
  Stuck Close/9(phi9) -> [phi9]
  Stuck Close/10(phi10) -> [phi10]
  Stuck Close/11(phi11) -> [phi11]
  Stuck Close/12(phi12) -> [phi12]
  Stuck Close/13(phi13) -> [phi13]
  Stuck Close/14(phi14) -> [phi14]

== system five_tank_hybrid_system/Scenarios/Stuck Close Valve 3 ==
  Fault_time : Constant  Value=180
  Stuck Close : Stateflow chart  TreatAsAtomicUnit=on
  tag scope: phi10=global, phi11=global, phi12=global, phi13=global, phi14=global, phi15=global, phi16=global, phi1=global, phi2=global, phi3=global, phi4=global, phi5=global, phi6=global, phi7=global, phi8=global, phi9=global
  wires:
  Stuck Close/14(phi14) -> [phi14]
  Stuck Close/13(phi13) -> [phi13]
  Stuck Close/12(phi12) -> [phi12]
  Stuck Close/11(phi11) -> [phi11]
  Stuck Close/10(phi10) -> [phi10]
  Stuck Close/9(phi9) -> [phi9]
  Stuck Close/8(phi8) -> [phi8]
  Stuck Close/7(phi7) -> [phi7]
  Stuck Close/6(phi6) -> [phi6]
  Stuck Close/5(phi5) -> [phi5]
  Stuck Close/4(phi4) -> [phi4]
  Stuck Close/3(phi3) -> [phi3]
  Stuck Close/2(phi2) -> [phi2]
  Stuck Close/1(phi1) -> [phi1]
  Stuck Close/15(phi15) -> [phi15]
  Stuck Close/16(phi16) -> [phi16]
  Fault_time/1 -> Stuck Close/1(Tf)

== system five_tank_hybrid_system/Scenarios/Stuck Close Valve 4 ==
  Fault_time : Constant  Value=320
  Stuck Close : Stateflow chart  TreatAsAtomicUnit=on
  tag scope: phi10=global, phi11=global, phi12=global, phi13=global, phi14=global, phi15=global, phi16=global, phi1=global, phi2=global, phi3=global, phi4=global, phi5=global, phi6=global, phi7=global, phi8=global, phi9=global
  wires:
  Fault_time/1 -> Stuck Close/1(Tf)
  Stuck Close/16(phi16) -> [phi16]
  Stuck Close/15(phi15) -> [phi15]
  Stuck Close/1(phi1) -> [phi1]
  Stuck Close/2(phi2) -> [phi2]
  Stuck Close/3(phi3) -> [phi3]
  Stuck Close/4(phi4) -> [phi4]
  Stuck Close/5(phi5) -> [phi5]
  Stuck Close/6(phi6) -> [phi6]
  Stuck Close/7(phi7) -> [phi7]
  Stuck Close/8(phi8) -> [phi8]
  Stuck Close/9(phi9) -> [phi9]
  Stuck Close/10(phi10) -> [phi10]
  Stuck Close/11(phi11) -> [phi11]
  Stuck Close/12(phi12) -> [phi12]
  Stuck Close/13(phi13) -> [phi13]
  Stuck Close/14(phi14) -> [phi14]

== system five_tank_hybrid_system/Scenarios/Stuck Open Valve 1 ==
  Fault_time : Constant  Value=150
  Stuck Open : Stateflow chart  TreatAsAtomicUnit=on
  tag scope: phi10=global, phi11=global, phi12=global, phi13=global, phi14=global, phi15=global, phi16=global, phi1=global, phi2=global, phi3=global, phi4=global, phi5=global, phi6=global, phi7=global, phi8=global, phi9=global
  wires:
  Fault_time/1 -> Stuck Open/1(Tf)
  Stuck Open/16(phi16) -> [phi16]
  Stuck Open/15(phi15) -> [phi15]
  Stuck Open/1(phi1) -> [phi1]
  Stuck Open/2(phi2) -> [phi2]
  Stuck Open/3(phi3) -> [phi3]
  Stuck Open/4(phi4) -> [phi4]
  Stuck Open/5(phi5) -> [phi5]
  Stuck Open/6(phi6) -> [phi6]
  Stuck Open/7(phi7) -> [phi7]
  Stuck Open/8(phi8) -> [phi8]
  Stuck Open/9(phi9) -> [phi9]
  Stuck Open/10(phi10) -> [phi10]
  Stuck Open/11(phi11) -> [phi11]
  Stuck Open/12(phi12) -> [phi12]
  Stuck Open/13(phi13) -> [phi13]
  Stuck Open/14(phi14) -> [phi14]

== system five_tank_hybrid_system/Scenarios/Stuck Open Valve 2 ==
  Fault_time : Constant  Value=200
  Stuck Open : Stateflow chart  TreatAsAtomicUnit=on
  tag scope: phi10=global, phi11=global, phi12=global, phi13=global, phi14=global, phi15=global, phi16=global, phi1=global, phi2=global, phi3=global, phi4=global, phi5=global, phi6=global, phi7=global, phi8=global, phi9=global
  wires:
  Stuck Open/14(phi14) -> [phi14]
  Stuck Open/13(phi13) -> [phi13]
  Stuck Open/12(phi12) -> [phi12]
  Stuck Open/11(phi11) -> [phi11]
  Stuck Open/10(phi10) -> [phi10]
  Stuck Open/9(phi9) -> [phi9]
  Stuck Open/8(phi8) -> [phi8]
  Stuck Open/7(phi7) -> [phi7]
  Stuck Open/6(phi6) -> [phi6]
  Stuck Open/5(phi5) -> [phi5]
  Stuck Open/4(phi4) -> [phi4]
  Stuck Open/3(phi3) -> [phi3]
  Stuck Open/2(phi2) -> [phi2]
  Stuck Open/1(phi1) -> [phi1]
  Stuck Open/15(phi15) -> [phi15]
  Stuck Open/16(phi16) -> [phi16]
  Fault_time/1 -> Stuck Open/1(Tf)

== system five_tank_hybrid_system/Scenarios/Stuck Open Valve 3 ==
  Fault_time : Constant  Value=400
  Stuck Open : Stateflow chart  TreatAsAtomicUnit=on
  tag scope: phi10=global, phi11=global, phi12=global, phi13=global, phi14=global, phi15=global, phi16=global, phi1=global, phi2=global, phi3=global, phi4=global, phi5=global, phi6=global, phi7=global, phi8=global, phi9=global
  wires:
  Fault_time/1 -> Stuck Open/1(Tf)
  Stuck Open/16(phi16) -> [phi16]
  Stuck Open/15(phi15) -> [phi15]
  Stuck Open/1(phi1) -> [phi1]
  Stuck Open/2(phi2) -> [phi2]
  Stuck Open/3(phi3) -> [phi3]
  Stuck Open/4(phi4) -> [phi4]
  Stuck Open/5(phi5) -> [phi5]
  Stuck Open/6(phi6) -> [phi6]
  Stuck Open/7(phi7) -> [phi7]
  Stuck Open/8(phi8) -> [phi8]
  Stuck Open/9(phi9) -> [phi9]
  Stuck Open/10(phi10) -> [phi10]
  Stuck Open/11(phi11) -> [phi11]
  Stuck Open/12(phi12) -> [phi12]
  Stuck Open/13(phi13) -> [phi13]
  Stuck Open/14(phi14) -> [phi14]

== system five_tank_hybrid_system/Scenarios/Stuck Open Valve 4 ==
  Fault_time : Constant  Value=450
  Stuck Open : Stateflow chart  TreatAsAtomicUnit=on
  tag scope: phi10=global, phi11=global, phi12=global, phi13=global, phi14=global, phi15=global, phi16=global, phi1=global, phi2=global, phi3=global, phi4=global, phi5=global, phi6=global, phi7=global, phi8=global, phi9=global
  wires:
  Stuck Open/14(phi14) -> [phi14]
  Stuck Open/13(phi13) -> [phi13]
  Stuck Open/12(phi12) -> [phi12]
  Stuck Open/11(phi11) -> [phi11]
  Stuck Open/10(phi10) -> [phi10]
  Stuck Open/9(phi9) -> [phi9]
  Stuck Open/8(phi8) -> [phi8]
  Stuck Open/7(phi7) -> [phi7]
  Stuck Open/6(phi6) -> [phi6]
  Stuck Open/5(phi5) -> [phi5]
  Stuck Open/4(phi4) -> [phi4]
  Stuck Open/3(phi3) -> [phi3]
  Stuck Open/2(phi2) -> [phi2]
  Stuck Open/1(phi1) -> [phi1]
  Stuck Open/15(phi15) -> [phi15]
  Stuck Open/16(phi16) -> [phi16]
  Fault_time/1 -> Stuck Open/1(Tf)

== stateflow chart five_tank_hybrid_system/A7_Pump2/Chart1 ==
  state Off
    entry: q=1;
  state On
    entry: q=2;
  state Fail
    entry: q=3;
  (default) -> Off
  Off -> On [order 1] : [x2<=X2min]
  On -> Off [order 1] : [x2>=X2max]
  Off -> Fail [order 2] : [phi7==1]
  On -> Fail [order 2] : [phi7==1]
  data: x2 input; phi7 input; q output; X2max parameter; X2min parameter

== stateflow chart five_tank_hybrid_system/A8_Pump3/Chart2 ==
  state Off
    entry: q=1;
  state On
    entry: q=2;
  state Fail
    entry: q=3;
  (default) -> Off
  Off -> On [order 1] : [x5<=X5min]
  On -> Off [order 1] : [x5>=X5max]
  Off -> Fail [order 2] : [phi8==1]
  On -> Fail [order 2] : [phi8==1]
  data: X5min parameter; X5max parameter; x5 input; phi8 input; q output

== stateflow chart five_tank_hybrid_system/A6_Pump1/Chart ==
  state Off
    entry: q=1;
  state On
    entry: q=2;
  state Fail
    entry: q=3;
  (default) -> Off
  Off -> On [order 1] : [x1<=X1min]
  On -> Off [order 1] : [x1>=X1max]
  Off -> Fail [order 2] : [phi6==1]
  On -> Fail [order 2] : [phi6==1]
  data: x1 input; X1min parameter; X1max parameter; phi6 input; q output

== stateflow chart five_tank_hybrid_system/A1_Tank1/Chart ==
  state Healthy
    entry: q=1;
  state Leak
    entry: q=2;
  (default) -> Healthy
  Healthy -> Leak : [phi==1]
  data: phi input; q output

== matlab function five_tank_hybrid_system/A1_Tank1/MATLAB Function ==
  data: zin input; x output; zout input; cp input; Ap input; A input; g input; x input
function x = fm(zin,zout,cp,Ap,A,g,x)

x = 1/A*(zin-zout-(cp*Ap*sqrt(2*g*x)));

== matlab function five_tank_hybrid_system/A1_Tank1/MATLAB Function1 ==
  data: A input; rho input; g input; x input; f1 output
function f1 = f_leak(A,rho,g,x)

f1 = -1/A*pi*rho^2*sqrt(2*g*x);

== stateflow chart five_tank_hybrid_system/A2_Tank2/Chart ==
  state Healthy
    entry: q=1;
  state Leak
    entry: q=2;
  (default) -> Healthy
  Healthy -> Leak : [phi==1]
  data: q output; phi input

== matlab function five_tank_hybrid_system/A2_Tank2/MATLAB Function ==
  data: zin input; x output; zout input; cp input; Ap input; A input; g input; x input
function x = fm(zin,zout,cp,Ap,A,g,x)

x = 1/A*(zin-zout-(cp*Ap*sqrt(2*g*x)));

== matlab function five_tank_hybrid_system/A2_Tank2/MATLAB Function1 ==
  data: A input; rho input; g input; x input; f1 output
function f1 = f_leak(A,rho,g,x)

f1 = -1/A*pi*rho^2*sqrt(2*g*x);

== stateflow chart five_tank_hybrid_system/A3_Tank3/Chart ==
  state Healthy
    entry: q=1;
  state Leak
    entry: q=2;
  (default) -> Healthy
  Healthy -> Leak : [phi==1]
  data: q output; phi input

== matlab function five_tank_hybrid_system/A3_Tank3/MATLAB Function ==
  data: zin input; x output; zout input; cp input; Ap input; A input; g input; x input
function x = fm(zin,zout,cp,Ap,A,g,x)

x = 1/A*(zin-zout-(cp*Ap*sqrt(2*g*x)));

== matlab function five_tank_hybrid_system/A3_Tank3/MATLAB Function1 ==
  data: A input; rho input; g input; x input; f1 output
function f1 = f_leak(A,rho,g,x)

f1 = -1/A*pi*rho^2*sqrt(2*g*x);

== stateflow chart five_tank_hybrid_system/A4_Tank4/Chart ==
  state Healthy
    entry: q=1;
  state Leak
    entry: q=2;
  (default) -> Healthy
  Healthy -> Leak : [phi==1]
  data: q output; phi input

== matlab function five_tank_hybrid_system/A4_Tank4/MATLAB Function ==
  data: zin input; x output; zout input; cp input; Ap input; A input; g input; x input
function x = fm(zin,zout,cp,Ap,A,g,x)

x = 1/A*(zin-zout-(cp*Ap*sqrt(2*g*x)));

== matlab function five_tank_hybrid_system/A4_Tank4/MATLAB Function1 ==
  data: A input; rho input; g input; x input; f1 output
function f1 = f_leak(A,rho,g,x)

f1 = -1/A*pi*rho^2*sqrt(2*g*x);

== stateflow chart five_tank_hybrid_system/A5_Tank5/Chart ==
  state Healthy
    entry: q=1;
  state Leak
    entry: q=2;
  (default) -> Healthy
  Healthy -> Leak : [phi==1]
  data: q output; phi input

== matlab function five_tank_hybrid_system/A5_Tank5/MATLAB Function ==
  data: zin input; x output; zout input; cp input; Ap input; A input; g input; x input
function x = fm(zin,zout,cp,Ap,A,g,x)

x = 1/A*(zin-zout-(cp*Ap*sqrt(2*g*x)));

== matlab function five_tank_hybrid_system/A5_Tank5/MATLAB Function1 ==
  data: A input; rho input; g input; x input; f1 output
function f1 = f_leak(A,rho,g,x)

f1 = -1/A*pi*rho^2*sqrt(2*g*x);

== stateflow chart five_tank_hybrid_system/A11_Valve3/Chart ==
  state Stuck_Open
    entry: q=4;
  state Close
    entry: q=1;
  state Open
    entry: q=2;
  state Stuck_Close
    entry: q=3;
  Close -> Stuck_Open [order 2] : [phi14==1]
  Open -> Stuck_Open [order 2] : [phi14==1]
  (default) -> Close
  Close -> Open [order 1] : [u1==1]
  Open -> Close [order 1] : [u1==0]
  Close -> Stuck_Close [order 3] : [phi13==1]
  Open -> Stuck_Close [order 3] : [phi13==1]
  data: u1 input; phi13 input; phi14 input; q output

== matlab function five_tank_hybrid_system/A11_Valve3/MATLAB Function ==
  data: cv input; z output; Av input; in1 input; in2 input; g input
function z = fm(cv,Av,in1,in2,g)

z = cv*Av*sign(in1-in2)*sqrt(2*g*abs(in1-in2));

== stateflow chart five_tank_hybrid_system/A12_Valve4/Chart ==
  state Stuck_Open
    entry: q=4;
  state Close
    entry: q=1;
  state Open
    entry: q=2;
  state Stuck_Close
    entry: q=3;
  Close -> Stuck_Open [order 2] : [phi16==1]
  Open -> Stuck_Open [order 2] : [phi16==1]
  (default) -> Close
  Close -> Open [order 1] : [u2==1]
  Open -> Close [order 1] : [u2==0]
  Close -> Stuck_Close [order 3] : [phi15==1]
  Open -> Stuck_Close [order 3] : [phi15==1]
  data: u2 input; phi15 input; phi16 input; q output

== matlab function five_tank_hybrid_system/A12_Valve4/MATLAB Function ==
  data: cv input; z output; Av input; in1 input; in2 input; g input
function z = fm(cv,Av,in1,in2,g)

z = cv*Av*sign(in1-in2)*sqrt(2*g*abs(in1-in2));
